simulink model "Task2"  (R2019a)
settings: Solver=VariableStepAuto  StartTime=0.0  StopTime=50  RelTol=1e-3
libraries: fl_lib x13, nesl_utility x4, simulink_extras x2, sdl_lib x1
settings Model: Creator=hp  LastModifiedBy=hp

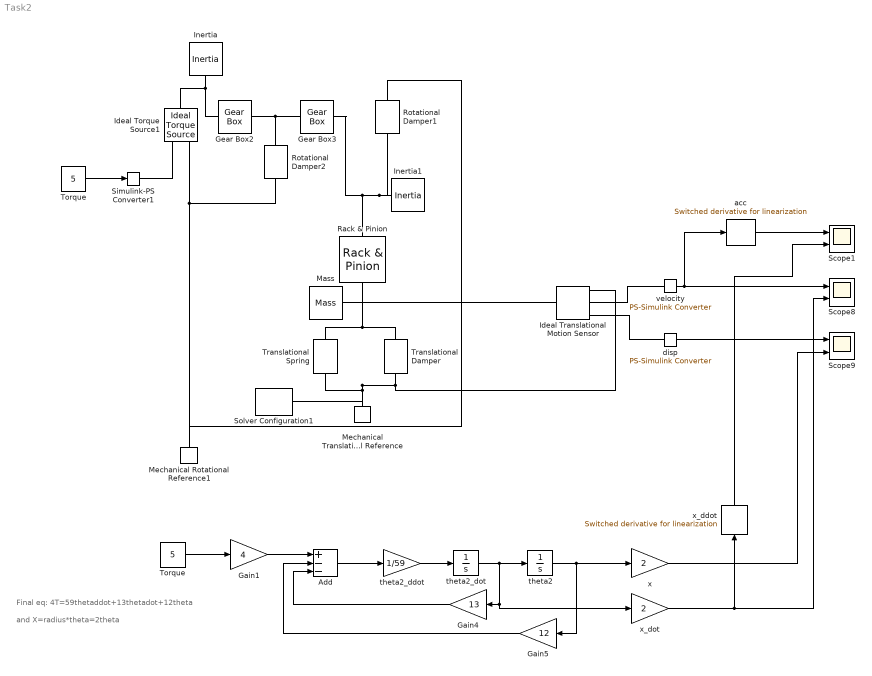
== system Task2 ==
  note: and X=radius*theta=2theta
  note: Final eq: 4T=59thetaddot+13thetadot+12theta
  Add : Sum  Inputs=+--
  Gain1 : Gain  Gain=4
  Gain4 : Gain  Gain=13
  Gain5 : Gain  Gain=12
  Gear Box2 : fl_lib/Mechanical/Mechanisms/Gear Box  ratio=2  t_in_specify=off  t_in_priority=None  t_in=0 N*m  t_in_nominal_specify=off  t_in_nominal_unit=N*m  t_in_nominal_value=1  t_out_specify=off  t_out_priority=None  t_out=0 N*m  t_out_nominal_specify=off  t_out_nominal_unit=N*m  t_out_nominal_value=1
  Gear Box3 : fl_lib/Mechanical/Mechanisms/Gear Box  ratio=2  t_in_specify=off  t_in_priority=None  t_in=0 N*m  t_in_nominal_specify=off  t_in_nominal_unit=N*m  t_in_nominal_value=1  t_out_specify=off  t_out_priority=None  t_out=0 N*m  t_out_nominal_specify=off  t_out_nominal_unit=N*m  t_out_nominal_value=1
  Ideal Torque Source1 : fl_lib/Mechanical/Mechanical Sources/Ideal Torque Source
  Ideal Translational Motion Sensor : fl_lib/Mechanical/Mechanical Sensors/Ideal Translational Motion Sensor  offset=0 m
  Inertia : fl_lib/Mechanical/Rotational Elements/Inertia  inertia=3 kg*m^2  w_specify=off  w_priority=High  w=0 rad/s  w_nominal_specify=off  w_nominal_unit=rad/s  w_nominal_value=1  t_specify=off  t_priority=None  t=0 N*m  t_nominal_specify=off  t_nominal_unit=N*m  t_nominal_value=1
  Inertia1 : fl_lib/Mechanical/Rotational Elements/Inertia  inertia=3 kg*m^2  w_specify=off  w_priority=High  w=0 rad/s  w_nominal_specify=off  w_nominal_unit=rad/s  w_nominal_value=1  t_specify=off  t_priority=None  t=0 N*m  t_nominal_specify=off  t_nominal_unit=N*m  t_nominal_value=1
  Mass : fl_lib/Mechanical/Translational Elements/Mass  mass=2 kg  v_specify=off  v_priority=High  v=0 m/s  v_nominal_specify=off  v_nominal_unit=m/s  v_nominal_value=1  f_specify=off  f_priority=None  f=0 N  f_nominal_specify=off  f_nominal_unit=N  f_nominal_value=1
  Mechanical Rotational Reference1 : fl_lib/Mechanical/Rotational Elements/Mechanical Rotational Reference
  Mechanical Translational Reference : fl_lib/Mechanical/Translational Elements/Mechanical Translational Reference
  Rack & Pinion : sdl_lib/Gears/Rotational- Translational/Rack & Pinion  param=1  radius=2 m  n_teeth=20  x_tooth=5 mm  rack_direction_sign=1  friction_model=1  efficiency=0.8  mu_visc_P=0 N*m/(rad/s)  mu_visc_R=0 N/(m/s)  pwr_thr=0.001 W  temperature_TLU=[280, 300, 320] K  efficiency_TLU=[.95, .9, .85]  thermal_mass=50 J/K  T_init=300 K
      settings: SourceProductName=Simscape Driveline  SourceProductBaseCode=LD
  Rotational Damper1 : fl_lib/Mechanical/Rotational Elements/Rotational Damper  D=1 N*m/(rad/s)  w_specify=off  w_priority=None  w=0 rad/s  w_nominal_specify=off  w_nominal_unit=rad/s  w_nominal_value=1  t_specify=off  t_priority=None  t=0 N*m  t_nominal_specify=off  t_nominal_unit=N*m  t_nominal_value=1
  Rotational Damper2 : fl_lib/Mechanical/Rotational Elements/Rotational Damper  D=1 N*m/(rad/s)  w_specify=off  w_priority=None  w=0 rad/s  w_nominal_specify=off  w_nominal_unit=rad/s  w_nominal_value=1  t_specify=off  t_priority=None  t=0 N*m  t_nominal_specify=off  t_nominal_unit=N*m  t_nominal_value=1
  Scope1 : Scope  NumInputPorts=2
  Scope8 : Scope  NumInputPorts=2
  Scope9 : Scope  NumInputPorts=2
  Simulink-PS Converter1 : nesl_utility/Simulink-PS Converter  PhysicalDomain=network_engine_domain  SubClassName=ps_input  LeftPortType=input  RightPortType=output  PseudoPeriodic=off  Frequencies=[]  NoiseDistribution=none  NoiseParameters=[]  Unit=1  AffineConversion=off  FilteringAndDerivatives=provide  SimscapeFilterOrder=1  InputFilterTimeConstant=0.001  UdotUserProvided=0
  Solver Configuration1 : nesl_utility/Solver Configuration  PhysicalDomain=network_engine_domain  SubClassName=solver  LeftPortType=input  RightPortType=generic  Tones=[]  Harmonics=[]  SimulateNoise=off  Profile=off  UseLocalSampling=off  EnableSwitchedLinearOptims=on  FrequencyDomain=off  UseCCode=off  RelTol=0.001  AbsTol=1e-06  MinStep=1e-09  ToWorkspace=off  RevertToSquareIcSolve=off  NumHomotopyIterations=100  PhasorMode=off  PhasorModeNumHarmonics=1  DoDC=off  ResidualTolerance=1e-09  UseLocalSolver=off  LocalSolverChoice=NE_BACKWARD_EULER_ADVANCER  LocalSolverSampleTime=0.001  DoFixedCost=off  MaxNonlinIter=3  MaxModeIter=2  LinearAlgebra=auto  EquationFormulation=NE_TIME_EF  DelaysMemoryBudget=1024  AutomaticFiltering=on  FilteringTimeConstant=0.001  PartitionStorageMethod=AS_NEEDED  PartitionMemoryBudget=1024  PartitionMethod=ROBUST
  Torque : Constant  Value=5
  "Torque " : Constant  Value=5
  Translational Damper : fl_lib/Mechanical/Translational Elements/Translational Damper  D=2 N/(m/s)  v_specify=off  v_priority=None  v=0 m/s  v_nominal_specify=off  v_nominal_unit=m/s  v_nominal_value=1  f_specify=off  f_priority=None  f=0 N  f_nominal_specify=off  f_nominal_unit=N  f_nominal_value=1
  Translational Spring : fl_lib/Mechanical/Translational Elements/Translational Spring  spr_rate=3 N/m  v_specify=off  v_priority=None  v=0 m/s  v_nominal_specify=off  v_nominal_unit=m/s  v_nominal_value=1  f_specify=off  f_priority=None  f=0 N  f_nominal_specify=off  f_nominal_unit=N  f_nominal_value=1  x_specify=off  x_priority=High  x=0 m  x_nominal_specify=off  x_nominal_unit=m  x_nominal_value=1
  acc : simulink_extras/Linearization/Switched derivative for linearization  switchVal=0  derivConst=100
      settings: SourceProductName=Simulink  SourceProductBaseCode=SL
  disp : nesl_utility/PS-Simulink Converter  PhysicalDomain=network_engine_domain  SubClassName=ps_output  LeftPortType=input  RightPortType=output  PseudoPeriodic=off  Frequencies=[]  Unit=1  AffineConversion=off
  theta2 : Integrator
  theta2_ddot : Gain  Gain=1/59
  theta2_dot : Integrator
  velocity : nesl_utility/PS-Simulink Converter  PhysicalDomain=network_engine_domain  SubClassName=ps_output  LeftPortType=input  RightPortType=output  PseudoPeriodic=off  Frequencies=[]  Unit=1  AffineConversion=off
  x : Gain  Gain=2
  x_ddot : simulink_extras/Linearization/Switched derivative for linearization  switchVal=0  derivConst=100
      settings: SourceProductName=Simulink  SourceProductBaseCode=SL
  x_dot : Gain  Gain=2
  wires:
  Add/1 -> theta2_ddot/1
  "Torque "/1 -> Gain1/1
  velocity/1 -> acc/1, Scope8/1
  Torque/1 -> Simulink-PS Converter1/1
  disp/1 -> Scope9/1
  theta2_ddot/1 -> theta2_dot/1
  theta2_dot/1 -> x_dot/1, Gain4/1, theta2/1
  Gain4/1 -> Add/3
  theta2/1 -> x/1, Gain5/1
  Gain5/1 -> Add/2
  x/1 -> Scope9/2
  x_dot/1 -> x_ddot/1, Scope8/2
  acc/1 -> Scope1/1
  x_ddot/1 -> Scope1/2
  Gain1/1 -> Add/1
  connections:
  Ideal Torque Source1/LConn1 -- Gear Box2/LConn1 -- Inertia/LConn1
  Translational Damper/RConn1 -- Solver Configuration1/RConn1 -- Mechanical Translational Reference/LConn1 -- Translational Spring/RConn1 -- Ideal Translational Motion Sensor/RConn1
  Rotational Damper1/RConn1 -- Mechanical Rotational Reference1/LConn1 -- Rotational Damper2/RConn1 -- Ideal Torque Source1/RConn2
  Translational Damper/LConn1 -- Ideal Translational Motion Sensor/LConn1 -- Rack & Pinion/RConn1 -- Mass/LConn1 -- Translational Spring/LConn1
  Simulink-PS Converter1/RConn1 -- Ideal Torque Source1/RConn1
  Ideal Translational Motion Sensor/RConn2 -- velocity/LConn1
  Ideal Translational Motion Sensor/RConn3 -- disp/LConn1
  Rotational Damper2/LConn1 -- Gear Box2/RConn1 -- Gear Box3/LConn1
  Inertia1/LConn1 -- Rack & Pinion/LConn1 -- Gear Box3/RConn1 -- Rotational Damper1/LConn1
